simulink model "gm_test_prediction_without_delays"  (R2022a)
settings: Solver=FixedStepDiscrete  StartTime=0.0  StopTime=10.0  RelTol=1e-3
undefined symbols (not defined in the file or in its folder): f_c, L_d, L_q, L_x, L_y, p, psi_pm, R_ph
libraries: hdlmdlgenlib x2
(part 9 of 9)

== system gm_test_prediction_without_delays/Prediction_and_cost_function1/Subsystem/Subsystem9/Product11 ==
  In1 : Inport
  In2 : Inport  Port=2
  Product11 : Product  Inputs=**  OutDataTypeStr=single  SampleTime=1e-08
  Product11_pd1 : Delay  DelayLength=6
  Out1 : Outport
  wires:
  In1/1 -> Product11/1
  In2/1 -> Product11/2
  Product11/1 -> Product11_pd1/1
  Product11_pd1/1 -> Out1/1

== system gm_test_prediction_without_delays/Prediction_and_cost_function1/Subsystem/Subsystem9/Product2 ==
  In1 : Inport
  In2 : Inport  Port=2
  Product2 : Product  Inputs=**  OutDataTypeStr=single  SampleTime=1e-08
  Product2_pd1 : Delay  DelayLength=6
  Out1 : Outport
  wires:
  In1/1 -> Product2/1
  In2/1 -> Product2/2
  Product2/1 -> Product2_pd1/1
  Product2_pd1/1 -> Out1/1

== system gm_test_prediction_without_delays/Prediction_and_cost_function1/Subsystem/Subsystem9/Product3 ==
  In1 : Inport
  In2 : Inport  Port=2
  Product3 : Product  Inputs=**  OutDataTypeStr=single  SampleTime=1e-08
  Product3_pd1 : Delay  DelayLength=6
  Out1 : Outport
  wires:
  In1/1 -> Product3/1
  In2/1 -> Product3/2
  Product3/1 -> Product3_pd1/1
  Product3_pd1/1 -> Out1/1

== system gm_test_prediction_without_delays/Prediction_and_cost_function1/Subsystem/Subsystem9/Product31 ==
  In1 : Inport
  In2 : Inport  Port=2
  Product31 : Product  Inputs=**  OutDataTypeStr=single  SampleTime=1e-08
  Product31_pd1 : Delay  DelayLength=6
  Out1 : Outport
  wires:
  In1/1 -> Product31/1
  In2/1 -> Product31/2
  Product31/1 -> Product31_pd1/1
  Product31_pd1/1 -> Out1/1

== system gm_test_prediction_without_delays/Prediction_and_cost_function1/Subsystem/Subsystem9/Product4 ==
  In1 : Inport
  In2 : Inport  Port=2
  Product4 : Product  Inputs=**  OutDataTypeStr=single  SampleTime=1e-08
  Product4_pd1 : Delay  DelayLength=6
  Out1 : Outport
  wires:
  In1/1 -> Product4/1
  In2/1 -> Product4/2
  Product4/1 -> Product4_pd1/1
  Product4_pd1/1 -> Out1/1

== system gm_test_prediction_without_delays/Prediction_and_cost_function1/Subsystem/Subsystem9/Product5 ==
  In1 : Inport
  In2 : Inport  Port=2
  Product5 : Product  Inputs=**  OutDataTypeStr=single  SampleTime=1e-08
  Product5_pd1 : Delay  DelayLength=6
  Out1 : Outport
  wires:
  In1/1 -> Product5/1
  In2/1 -> Product5/2
  Product5/1 -> Product5_pd1/1
  Product5_pd1/1 -> Out1/1

== system gm_test_prediction_without_delays/Prediction_and_cost_function1/Subsystem/Subsystem9/Product6 ==
  In1 : Inport
  In2 : Inport  Port=2
  Product6 : Product  Inputs=**  OutDataTypeStr=single  SampleTime=1e-08
  Product6_pd1 : Delay  DelayLength=6
  Out1 : Outport
  wires:
  In1/1 -> Product6/1
  In2/1 -> Product6/2
  Product6/1 -> Product6_pd1/1
  Product6_pd1/1 -> Out1/1

== system gm_test_prediction_without_delays/Prediction_and_cost_function1/Subsystem/Subsystem9/Product7 ==
  In1 : Inport
  In2 : Inport  Port=2
  Product7 : Product  Inputs=**  OutDataTypeStr=single  SampleTime=1e-08
  Product7_pd1 : Delay  DelayLength=6
  Out1 : Outport
  wires:
  In1/1 -> Product7/1
  In2/1 -> Product7/2
  Product7/1 -> Product7_pd1/1
  Product7_pd1/1 -> Out1/1

== system gm_test_prediction_without_delays/Prediction_and_cost_function1/Subsystem/Subsystem9/Product8 ==
  In1 : Inport
  In2 : Inport  Port=2
  Product8 : Product  Inputs=**  OutDataTypeStr=single  SampleTime=1e-08
  Product8_pd1 : Delay  DelayLength=6
  Out1 : Outport
  wires:
  In1/1 -> Product8/1
  In2/1 -> Product8/2
  Product8/1 -> Product8_pd1/1
  Product8_pd1/1 -> Out1/1

== system gm_test_prediction_without_delays/Prediction_and_cost_function1/Subsystem/Subsystem9/Product9 ==
  In1 : Inport
  In2 : Inport  Port=2
  Product9 : Product  Inputs=**  OutDataTypeStr=single  SampleTime=1e-08
  Product9_pd1 : Delay  DelayLength=6
  Out1 : Outport
  wires:
  In1/1 -> Product9/1
  In2/1 -> Product9/2
  Product9/1 -> Product9_pd1/1
  Product9_pd1/1 -> Out1/1

== system gm_test_prediction_without_delays/Prediction_and_cost_function1/Subsystem/Subsystem9/Subtract1_stage2 ==
  In1 : Inport
  In2 : Inport  Port=2
  Subtract1_stage2 : Sum  Inputs=+-  OutDataTypeStr=single  SampleTime=1e-08
  Subtract1_stage2_pd1 : Delay  DelayLength=6
  Out1 : Outport
  wires:
  In1/1 -> Subtract1_stage2/1
  In2/1 -> Subtract1_stage2/2
  Subtract1_stage2/1 -> Subtract1_stage2_pd1/1
  Subtract1_stage2_pd1/1 -> Out1/1

== system gm_test_prediction_without_delays/Prediction_and_cost_function1/Subsystem/Subsystem9/Subtract1_stage3 ==
  In1 : Inport
  In2 : Inport  Port=2
  Subtract1_stage3 : Sum  Inputs=+-  OutDataTypeStr=single  SampleTime=1e-08
  Subtract1_stage3_pd1 : Delay  DelayLength=6
  Out1 : Outport
  wires:
  In1/1 -> Subtract1_stage3/1
  In2/1 -> Subtract1_stage3/2
  Subtract1_stage3/1 -> Subtract1_stage3_pd1/1
  Subtract1_stage3_pd1/1 -> Out1/1

== system gm_test_prediction_without_delays/Prediction_and_cost_function1/Subsystem/Subsystem9/Subtract2 ==
  In1 : Inport
  In2 : Inport  Port=2
  Subtract2 : Sum  Inputs=+-  OutDataTypeStr=single  SampleTime=1e-08
  Subtract2_pd1 : Delay  DelayLength=6
  Out1 : Outport
  wires:
  In1/1 -> Subtract2/1
  In2/1 -> Subtract2/2
  Subtract2/1 -> Subtract2_pd1/1
  Subtract2_pd1/1 -> Out1/1

== system gm_test_prediction_without_delays/Prediction_and_cost_function1/Subsystem/Subsystem9/Subtract3 ==
  In1 : Inport
  In2 : Inport  Port=2
  Subtract3 : Sum  Inputs=+-  OutDataTypeStr=single  SampleTime=1e-08
  Subtract3_pd1 : Delay  DelayLength=6
  Out1 : Outport
  wires:
  In1/1 -> Subtract3/1
  In2/1 -> Subtract3/2
  Subtract3/1 -> Subtract3_pd1/1
  Subtract3_pd1/1 -> Out1/1

== system gm_test_prediction_without_delays/Prediction_and_cost_function1/Subsystem/Subsystem9/Subtract_stage2 ==
  In1 : Inport
  In2 : Inport  Port=2
  Subtract_stage2 : Sum  Inputs=+-  OutDataTypeStr=single  SampleTime=1e-08
  Subtract_stage2_pd1 : Delay  DelayLength=6
  Out1 : Outport
  wires:
  In1/1 -> Subtract_stage2/1
  In2/1 -> Subtract_stage2/2
  Subtract_stage2/1 -> Subtract_stage2_pd1/1
  Subtract_stage2_pd1/1 -> Out1/1

== system gm_test_prediction_without_delays/Prediction_and_cost_function1/Subsystem/Subsystem9/Subtract_stage3 ==
  In1 : Inport
  In2 : Inport  Port=2
  Subtract_stage3 : Sum  OutDataTypeStr=single  SampleTime=1e-08
  Subtract_stage3_pd1 : Delay  DelayLength=6
  Out1 : Outport
  wires:
  In1/1 -> Subtract_stage3/1
  In2/1 -> Subtract_stage3/2
  Subtract_stage3/1 -> Subtract_stage3_pd1/1
  Subtract_stage3_pd1/1 -> Out1/1
